simulink model "sixscheme"  (R2022a)
settings: Solver=VariableStepAuto  StartTime=0.0  StopTime=0.128  RelTol=1e-3
libraries: commrandsrc3 x2, commseqgen3 x1
settings Model: Creator=Admin  LastModifiedBy=Admin

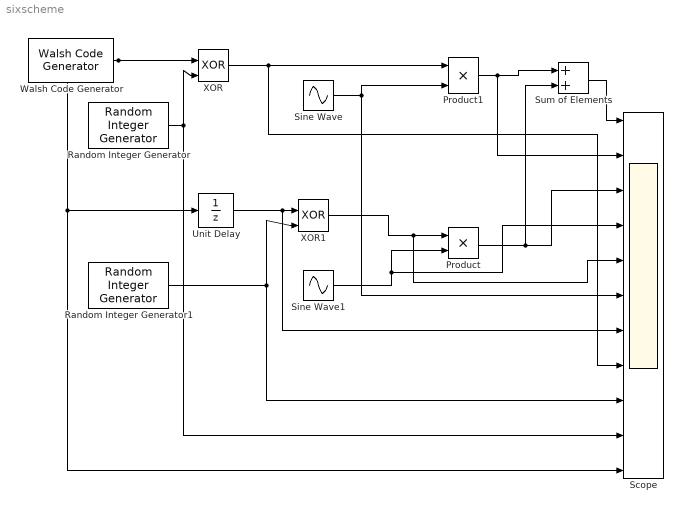
== system sixscheme ==
  Product : Product
  Product1 : Product
  Random Integer Generator : commrandsrc3/Random Integer Generator  SetSize=8  SeedSource=Parameter  Seed=01002  SampleTime=1/1.2288/10^6  SamplesPerFrame=1  OutputDataType=double  SimulateUsing=Interpreted execution
  Random Integer Generator1 : commrandsrc3/Random Integer Generator  SetSize=8  SeedSource=Auto  Seed=0  SampleTime=1/1.2288/10^6  SamplesPerFrame=1  OutputDataType=double  SimulateUsing=Interpreted execution
  Scope : Scope  NumInputPorts=11
  Sine Wave : Sin  SampleTime=0
  Sine Wave1 : Sin  SampleTime=0
  Sum of Elements : Sum
  Unit Delay : UnitDelay  SampleTime=-1  HasFrameUpgradeWarning=on
  Walsh Code Generator : commseqgen3/Walsh Code Generator  Length=64  Index=02  SampleTime=1/1.2288/10^6  SamplesPerFrame=1  OutputDataType=double  SimulateUsing=Code generation
      settings: SourceProductBaseCode=CM
  XOR : Logic  Operator=XOR  IconShape=distinctive  AllPortsSameDT=off  OutDataTypeStr=boolean
  XOR1 : Logic  Operator=XOR  IconShape=distinctive  AllPortsSameDT=off  OutDataTypeStr=boolean
  wires:
  Walsh Code Generator/1 -> XOR/1, Unit Delay/1, Scope/11
  Unit Delay/1 -> Scope/7, XOR1/1
  Random Integer Generator/1 -> Scope/10, XOR/2
  Random Integer Generator1/1 -> XOR1/2, Scope/9
  Sine Wave1/1 -> Scope/4, Product/2
  XOR1/1 -> Scope/5, Product/1
  Product/1 -> Sum of Elements/2, Scope/3
  Sine Wave/1 -> Product1/2, Scope/6
  XOR/1 -> Scope/8, Product1/1
  Product1/1 -> Scope/2, Sum of Elements/1
  Sum of Elements/1 -> Scope/1
